simulink model "Copy_of_bike_model_2states_smithFullBike"  (R2018b)
settings: Solver=VariableStepAuto  StartTime=0.0  StopTime=sim_time  FixedStep=Ts/10  MaxStep=Ts/10
values from neighbouring files (symbols this model uses):
  A_bike = [0 g/h_real ; 1 0]    [configuration.m]
  B_bike = [1 ; 0]    [configuration.m]
  b_compFilter = 1.095    [configuration.m]    (also in configuration_pidTuning.m)
  b_real = 1.095    [configuration.m]    (also in configuration_pidTuning.m)
  C1_bike = a_real/(b_real*h_real)    (= 0.392543973584)    [configuration.m]
  C2_bike = 1/(b_real*h_real)    (= 1.15454109878)    [configuration.m]
  C_ini = [C1_bike*input_velocity C2_bike*input_velocity^2]    [configuration.m]
  complementary = 0.985    [configuration.m]    (also in configuration_pidTuning.m)
  D = zeros(3,1)    [configuration_pidTuning.m]
  D_steering_position = 0.0    (= 0)    [configuration.m]
  delay_tf_steering = 0    [configuration.m]
  den_tf_steering = [1 245.9 0]    [configuration.m]
  den_tf_steering_dis = [den_tf_steering_dis 0] - [0 den_tf_steering_dis]    [configuration.m]
  direct_control = 1    [configuration.m]    (also in configuration_pidTuning.m)
  f_filter_phidot = 20    [configuration.m]
  filter_model = 1    [configuration.m]    (also in configuration_pidTuning.m)
  forward_motor_dynamics = 0    [configuration.m]    (also in configuration_pidTuning.m)
  forward_speed_offset = 0    [configuration.m]
  g = 9.81    [configuration.m]    (also in configuration_pidTuning.m)
  I_direct = 0.000227125326188444    (= 0.000227125326188)    [configuration.m]    (also in configuration_pidTuning.m)
  I_lat = 0.000115580509653549    (= 0.000115580509654)    [configuration.m]    (also in configuration_pidTuning.m)
  I_steering_position = 1    [configuration.m]    (also in simulate_bike.m = 30)
  IMU_height_model = 0.45    [configuration.m]    (also in configuration_pidTuning.m)
  IMU_height_real = 0.45    [configuration.m]    (also in configuration_pidTuning.m)
  initial_states = [deg2rad(-2) deg2rad(0) deg2rad(0)]    [configuration.m]    (also in configuration_pidTuning.m)
  input_velocity = 4    [configuration.m]    (also in configuration_pidTuning.m = 3)
  K_fullbike = 1    [configuration.m]
  lambda_compFilter = deg2rad(70)    [configuration.m]    (also in configuration_pidTuning.m)
  lambda_real = deg2rad(70)    [configuration.m]    (also in configuration_pidTuning.m)
  lat_control = 0    [configuration.m]    (also in configuration_pidTuning.m = 1)
  look_ahead = 0    [configuration.m]    (also in configuration_pidTuning.m)
  lqr_gains = zeros(length(velocity_lqr),1+size(A_bike,1))    [lqr_design.m]
  max_roll = pi/2    (= 1.57079632679)    [configuration.m]    (also in configuration_pidTuning.m)
  max_steering_motor_speed = 0.9    [configuration.m]    (also in configuration_pidTuning.m = 7.5)
  min_roll = - max_roll    (= -1.57079632679)    [configuration.m]    (also in configuration_pidTuning.m)
  min_steering_motor_speed = -0.9    [configuration.m]    (also in configuration_pidTuning.m = -7.5)
  noise = 0    [configuration.m]    (also in configuration_pidTuning.m)
  noise_acc = 2.4869e-05    [configuration.m]    (also in configuration_pidTuning.m)
  noise_encoder = 1e-7    (= 1e-07)    [configuration.m]    (also in configuration_pidTuning.m)
  noise_gyro = 0.005    [configuration.m]    (also in configuration_pidTuning.m = 0.0022)
  noise_hall = 0.0031    [configuration.m]    (also in configuration_pidTuning.m)
  noise_pos_meas = 0    [configuration.m]    (also in configuration_pidTuning.m = 0.51)
  num_tf_steering = [253.4]    [configuration.m]
  num_tf_steering_dis = [num_tf_steering_dis 0]    [configuration.m]
  offset_acc = 0.0*g    (= 0)    [configuration.m]
  offset_encoder = deg2rad(1)    [configuration.m]
  offset_gyro = deg2rad(0)    [configuration.m]
  offset_hall = 0.0    (= 0)    [configuration.m]
  offset_pos_x = 0    [configuration.m]
  offset_pos_y = 0    [configuration.m]
  P_direct = 0.0712859744206787    (= 0.0712859744207)    [configuration.m]    (also in configuration_pidTuning.m)
  P_lat = 0.0465435246389258    (= 0.0465435246389)    [configuration.m]    (also in configuration_pidTuning.m)
  P_steering_position = 10    [configuration.m]    (also in simulate_bike.m = 30)
  parameters_compFilter = [g h_compFilter b_compFilter a_compFilter lambda_compFilter c_compFilter]    [configuration.m]    (also in configuration_pidTuning.m)
  roll_rate_coef = 0.9    [configuration.m]    (also in configuration_pidTuning.m)
  sensor_offset = 0    [configuration.m]
  smith_fullbike = 1    [configuration.m]
  smith_steering = 0    [configuration.m]
  steering_angle_correction = deg2rad(0)    [configuration.m]
  sys_con = ss(A_lqr,B_lqr,C_lqr,D_lqr)    [lqr_design.m]
  time_offset_acc = 7    [configuration.m]
  time_offset_encoder = 10    [configuration.m]
  time_offset_gyro = 7    [configuration.m]
  time_offset_hall = 7    [configuration.m]
  time_offset_pos_x = 7    [configuration.m]
  time_offset_pos_y = 7    [configuration.m]
  Ts = 0.01    [configuration.m]    (also in configuration_pidTuning.m = 0.04)
  Ts_IMU = 0.01    [configuration.m]    (also in configuration_pidTuning.m = 0.04)
  velocity_lqr = [input_velocity - 0.1 , input_velocity , input_velocity + 0.1]    [lqr_design.m]
undefined symbols (not defined in the file or in its folder): A, B, cumulative_dist_along_path, curvature, den_filter_phidot, initial_x, initial_y, num_filter_phidot, path_x, path_y
libraries: simulink x14, simulink_extras x3, dspsigops x2
(part 1 of 3)
settings Model: Creator=Boaz Ash  LastModifiedBy=maximef
settings DebuggingCC: UnconnectedInputMsg=none  UnconnectedOutputMsg=none  UnconnectedLineMsg=none  LibraryContextMissingDiagnostic=none
settings SFSimCC: SimUseLocalCustomCode=off
settings RTWCC: RTWUseLocalCustomCode=off

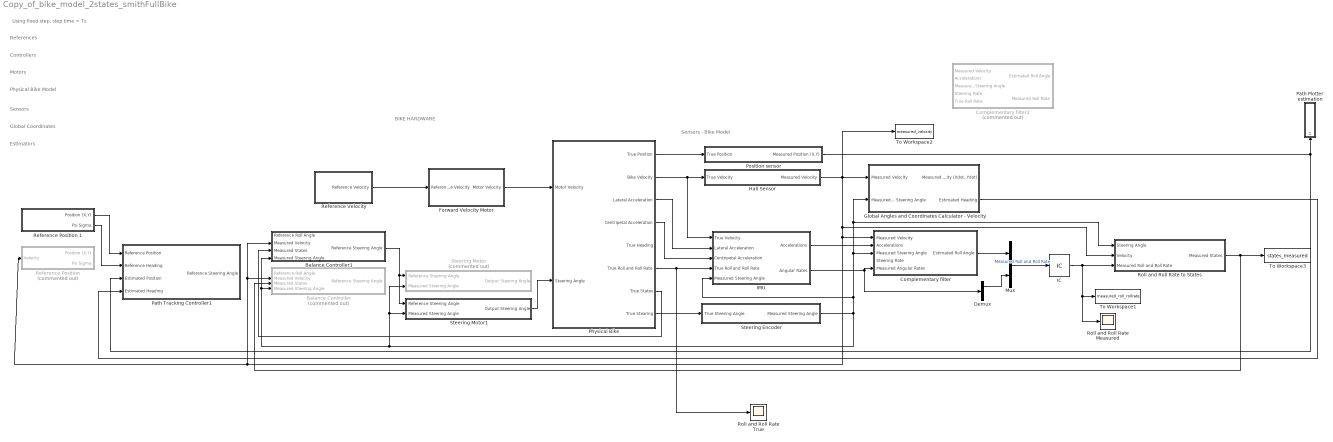
== system Copy_of_bike_model_2states_smithFullBike ==
  note: Using fixed step, step time = Ts
  note: BIKE HARDWARE
  note: References
  note: Physical Bike
      | Model
  note: Sensors - Bike Model
  note: Motors
  note: Sensors
  note: Global Coordinates
  note: Controllers
  note: Estimators
  Balance Controller : Subsystem  Commented=on  TreatAsAtomicUnit=on  SystemSampleTime=Ts
  Balance Controller1 : Subsystem  SystemSampleTime=Ts
  Complementary filter : Subsystem  SystemSampleTime=Ts_IMU
      settings: MinAlgLoopOccurrences=on
  Complementary filter2 : Subsystem  Commented=on  SystemSampleTime=Ts_IMU
      settings: MinAlgLoopOccurrences=on
  Demux : Demux  Outputs=3
  Forward Velocity Motor : Subsystem
  Global Angles and Coordinates Calculator - Velocity : Subsystem  SystemSampleTime=Ts
  Hall Sensor : Subsystem  TreatAsAtomicUnit=on  SystemSampleTime=Ts
  IC : InitialCondition  Value=[initial_states(1) initial_states(3)]'
  IMU : Subsystem  TreatAsAtomicUnit=on
  Mux : Mux  Inputs=2
  Path Plotter estimation : Subsystem  SystemSampleTime=Ts
  Path Tracking Controller1 : Subsystem
  Physical Bike : Subsystem
  Position sensor : Subsystem  TreatAsAtomicUnit=on  SystemSampleTime=Ts
  "Reference Position " : Subsystem  Commented=on
  Reference Position 1 : Subsystem
  "Reference Velocity " : Subsystem
  Roll and Roll Rate Measured : Scope
  Roll and Roll Rate True : Scope
  Roll and Roll Rate to States : Subsystem
  Steering Encoder : Subsystem  TreatAsAtomicUnit=on  SystemSampleTime=Ts
  Steering Motor : Subsystem  Commented=on
  Steering Motor1 : Subsystem
  To Workspace1 : ToWorkspace  VariableName=measured_roll_rollrate  SaveFormat=Timeseries  SampleTime=-1
  To Workspace2 : ToWorkspace  VariableName=measured_velocity  SaveFormat=Timeseries  SampleTime=-1
  To Workspace3 : ToWorkspace  VariableName=states_measured  SaveFormat=Timeseries  SampleTime=-1
  wires:
  "Reference Velocity "/1(Reference Velocity) -> Forward Velocity Motor/1(Reference Velocity)
  Forward Velocity Motor/1(Motor Velocity) -> Physical Bike/1(Motor Velocity)
  Position sensor/1("Measured Position (X,Y) ") -> Path Plotter estimation/1(Position), Path Tracking Controller1/3(Estimated Position)
  Global Angles and Coordinates Calculator - Velocity/2(Estimated Heading) -> Path Tracking Controller1/4(Estimated Heading)
  Physical Bike/3(Lateral Acceleration) -> IMU/2(Lateral Acceleration)
  Physical Bike/4(Centripetal Acceleration) -> IMU/3(Centripetal Acceleration)
  Steering Encoder/1(Measured Steering Angle) -> Steering Motor1/2(Measured Steering Angle), Steering Motor/2(Measured Steering Angle), Balance Controller1/4(Measured Steering Angle), Balance Controller/4(Measured Steering Angle), Roll and Roll Rate to States/1(Steering Angle), Global Angles and Coordinates Calculator - Velocity/2("Measured Steering Angle "), Complementary filter/3(Measured Steering Angle), IMU/5(Measured Steering Angle)
  IMU/1(Accelerations) -> Complementary filter/2(Accelerations)
  Hall Sensor/1(Measured Velocity) -> "Reference Position "/1(Velocity), Balance Controller1/2(Measured Velocity), Balance Controller/2(Measured Velocity), Complementary filter/1(Measured Velocity), Roll and Roll Rate to States/2(Velocity), To Workspace2/1, Global Angles and Coordinates Calculator - Velocity/1(Measured Velocity)
  Reference Position 1/2(Psi Sigma) -> Path Tracking Controller1/2(Reference Heading)
  Reference Position 1/1(Position (X,Y)) -> Path Tracking Controller1/1(Reference Position)
  Physical Bike/1(True Position) -> Position sensor/1(True Position)
  IMU/2(Angular Rates) -> Demux/1, Complementary filter/5(Measured Angular Rates)
  Physical Bike/8(True Stearing) -> Steering Encoder/1(True Steering Angle)
  Physical Bike/6(True Roll and Roll Rate) -> Roll and Roll Rate True/1, IMU/4(True Roll and Roll Rate)
  Physical Bike/2(Bike Velocity) -> IMU/1(True Velocity), Hall Sensor/1(True Velocity)
  IC/1 -> Roll and Roll Rate to States/3(Measured Roll and Roll Rate), Roll and Roll Rate Measured/1, To Workspace1/1
  Mux/1 -> IC/1  "Measured Roll and Roll Rate"
  Complementary filter/1(Estimated Roll Angle) -> Mux/1
  Demux/1 -> Mux/2
  Roll and Roll Rate to States/1(Measured States) -> Balance Controller/3(Measured States), To Workspace3/1
  Balance Controller1/1(Reference Steering Angle) -> Steering Motor1/1(Reference Steering Angle), Steering Motor/1(Reference Steering Angle)
  Physical Bike/7(True States) -> Balance Controller1/3(Measured States)
  Steering Motor1/1(Output Steering Angle) -> Physical Bike/2(Steering Angle)

== system Copy_of_bike_model_2states_smithFullBike/Balance Controller ==
  Reference Roll Angle : Inport
  Measured Velocity : Inport  Port=2
  Measured States : Inport  Port=3
  Measured Steering Angle : Inport  Port=4
  LQR Controller : Subsystem  TreatAsAtomicUnit=on  SystemSampleTime=Ts
  Mux : Mux  Inputs=2
  Reference States Generator : Subsystem  SystemSampleTime=Ts
  Sum : Sum  Inputs=|+-
  To Workspace : ToWorkspace  VariableName=states_measured  SaveFormat=Timeseries  SampleTime=-1
  Reference Steering Angle : Outport
  wires:
  Measured Velocity/1 -> LQR Controller/1(Velocity), Reference States Generator/1(Velocity)
  Measured States/1 -> To Workspace/1, Sum/2
  Measured Steering Angle/1 -> Reference States Generator/2(Steering Angle)
  Reference States Generator/1(State Error) -> LQR Controller/2(State Error)
  Sum/1 -> Reference States Generator/3(Angles Error)
  Mux/1 -> Sum/1
  Reference Roll Angle/1 -> Mux/1
  LQR Controller/1(Calculated Input) -> Reference Steering Angle/1

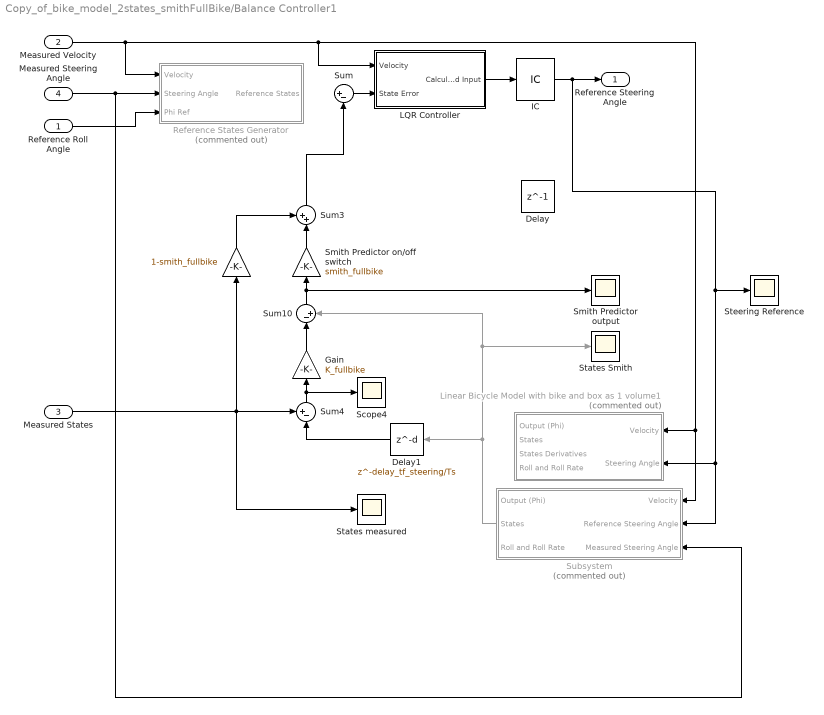
== system Copy_of_bike_model_2states_smithFullBike/Balance Controller1 ==
  Reference Roll Angle : Inport
  Measured Velocity : Inport  Port=2
  Measured States : Inport  Port=3
  Measured Steering Angle : Inport  Port=4
  " " : Gain  Gain=1-smith_fullbike
  Delay : Delay  DelayLength=1
  Delay1 : Delay  DelayLength=delay_tf_steering/Ts  SampleTime=Ts
  Gain : Gain  Gain=K_fullbike
  IC : InitialCondition  Value=0
  LQR Controller : Subsystem  TreatAsAtomicUnit=on  SystemSampleTime=Ts
  Linear Bicycle Model with bike and box as 1 volume1 : Subsystem  Commented=on
  Reference States Generator : Subsystem  Commented=on  SystemSampleTime=Ts
  Scope4 : Scope
  Smith Predictor on/off switch : Gain  Gain=smith_fullbike
  Smith Predictor output : Scope
  States Smith : Scope
  States measured : Scope
  Steering Reference : Scope
  Subsystem : Subsystem  Commented=on
  Sum : Sum  Inputs=|+-
  Sum10 : Sum  Inputs=|-+
  Sum3 : Sum  Inputs=++|
  Sum4 : Sum  Inputs=+-|
  Reference Steering Angle : Outport
  wires:
  Sum/1 -> LQR Controller/2(State Error)
  LQR Controller/1(Calculated Input) -> IC/1
  Reference Roll Angle/1 -> Reference States Generator/3(Phi Ref)
  Measured Steering Angle/1 -> Subsystem/3(Measured Steering Angle), Reference States Generator/2(Steering Angle)
  Measured States/1 -> " "/1, States measured/1, Sum4/1
  " "/1 -> Sum3/1
  Sum3/1 -> Sum/2
  Subsystem/2(States) -> Sum10/2, States Smith/1, Delay1/1
  Gain/1 -> Sum10/1
  Delay1/1 -> Sum4/2
  Smith Predictor on/off switch/1 -> Sum3/2
  Sum10/1 -> Smith Predictor output/1, Smith Predictor on/off switch/1
  Sum4/1 -> Scope4/1, Gain/1
  IC/1 -> Linear Bicycle Model with bike and box as 1 volume1/2(Steering Angle), Subsystem/2(Reference Steering Angle), Steering Reference/1, Reference Steering Angle/1
  Measured Velocity/1 -> Linear Bicycle Model with bike and box as 1 volume1/1(Velocity), Subsystem/1("Velocity "), LQR Controller/1(Velocity), Reference States Generator/1(Velocity)

== system Copy_of_bike_model_2states_smithFullBike/Complementary filter ==
  Measured Velocity : Inport
  Accelerations : Inport  Port=2
  Measured Steering Angle : Inport  Port=3
  Steering Rate : Inport  Port=4
  Measured Angular Rates : Inport  Port=5
  Complementary Filter : Subsystem  TreatAsAtomicUnit=on  SystemSampleTime=Ts_IMU
  Delay4 : Delay  DelayLength=1  SampleTime=Ts_IMU
  Demux : Demux  Outputs=3
  Downsample : DownSample  N=Ts/Ts_IMU  RateOptions=Allow multirate processing
  Roll Angle Estimation of Accelerometer : Subsystem
  To Workspace1 : ToWorkspace  VariableName=IMU_roll_angle  SaveFormat=Structure  SampleTime=-1
  Estimated Roll Angle : Outport
  wires:
  Roll Angle Estimation of Accelerometer/1(Roll Angle Estimation of Accelerometer) -> Complementary Filter/1(Roll Angle Estimation due to Accelerometer)  "Roll_acc"
  Complementary Filter/1(Roll Angle Estimation) -> Downsample/1, Delay4/1
  Measured Velocity/1 -> Roll Angle Estimation of Accelerometer/3(Measured Velocity)
  Measured Steering Angle/1 -> Roll Angle Estimation of Accelerometer/2(Measured Steering Angle)
  Steering Rate/1 -> Roll Angle Estimation of Accelerometer/4(Steering Rate)
  Demux/1 -> Roll Angle Estimation of Accelerometer/5(Roll Rate), Complementary Filter/2(Roll Rate due to Gyroscope)
  Accelerations/1 -> Roll Angle Estimation of Accelerometer/1(Accelerations)
  Measured Angular Rates/1 -> Demux/1
  Delay4/1 -> Roll Angle Estimation of Accelerometer/6(Measured Roll Angle)
  Downsample/1 -> Estimated Roll Angle/1, To Workspace1/1

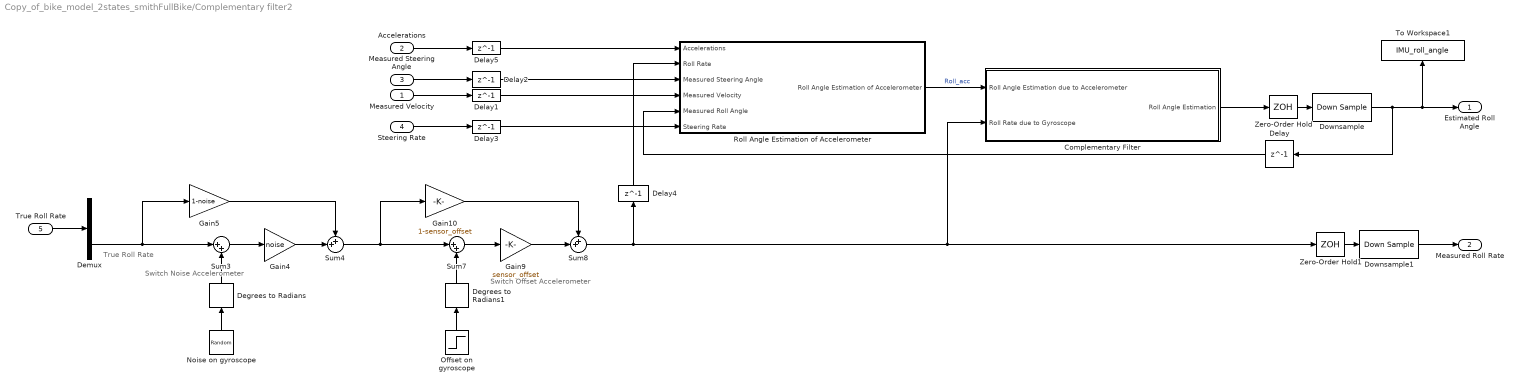
== system Copy_of_bike_model_2states_smithFullBike/Complementary filter2 ==
  note: Switch Noise
      | Accelerometer
  note: True Roll
      | Rate
  note: Switch Offset
      | Accelerometer
  Measured Velocity : Inport
  Accelerations : Inport  Port=2
  Measured Steering Angle : Inport  Port=3
  Steering Rate : Inport  Port=4
  True Roll Rate : Inport  Port=5
  Complementary Filter : Subsystem  TreatAsAtomicUnit=on  SystemSampleTime=Ts_IMU
  Degrees to Radians : simulink_extras/Transformations/Degrees to Radians
  Degrees to Radians1 : simulink_extras/Transformations/Degrees to Radians
  Delay{,1..2,4..5} (5 alike) : Delay  DelayLength=1
  Delay3 : Delay  DelayLength=1  SampleTime=Ts_IMU
  Demux : Demux  Outputs=2
  Downsample : DownSample  N=Ts/Ts_IMU  RateOptions=Allow multirate processing
  Downsample1 : DownSample  N=Ts/Ts_IMU  RateOptions=Allow multirate processing
  Gain10 : Gain  Gain=1-sensor_offset
  Gain4 : Gain  Gain=noise
  Gain5 : Gain  Gain=1-noise
  Gain9 : Gain  Gain=sensor_offset
  Noise on gyroscope : RandomNumber  Variance=noise_gyro  SampleTime=Ts
  Offset on gyroscope : Step  Time=time_offset_gyro  After=offset_gyro  SampleTime=Ts
  Roll Angle Estimation of Accelerometer : Subsystem
  Sum3 : Sum  Inputs=|++
  Sum4 : Sum  Inputs=++|
  Sum7 : Sum  Inputs=|++
  Sum8 : Sum  Inputs=++|
  To Workspace1 : ToWorkspace  VariableName=IMU_roll_angle  SaveFormat=Structure  SampleTime=-1
  Zero-Order Hold : ZeroOrderHold  SampleTime=Ts_IMU
  Zero-Order Hold1 : ZeroOrderHold  SampleTime=Ts_IMU
  Estimated Roll Angle : Outport
  Measured Roll Rate : Outport  Port=2
  wires:
  Roll Angle Estimation of Accelerometer/1(Roll Angle Estimation of Accelerometer) -> Complementary Filter/1(Roll Angle Estimation due to Accelerometer)  "Roll_acc"
  Sum8/1 -> Zero-Order Hold1/1, Complementary Filter/2(Roll Rate due to Gyroscope), Delay4/1
  Zero-Order Hold/1 -> Downsample/1
  Zero-Order Hold1/1 -> Downsample1/1
  Accelerations/1 -> Delay5/1
  Measured Steering Angle/1 -> Delay2/1
  Measured Velocity/1 -> Delay1/1
  Delay/1 -> Roll Angle Estimation of Accelerometer/5(Measured Roll Angle)
  Delay1/1 -> Roll Angle Estimation of Accelerometer/4(Measured Velocity)
  Delay2/1 -> Roll Angle Estimation of Accelerometer/3(Measured Steering Angle)
  Steering Rate/1 -> Delay3/1
  Delay3/1 -> Roll Angle Estimation of Accelerometer/6(Steering Rate)
  Delay4/1 -> Roll Angle Estimation of Accelerometer/2(Roll Rate)
  Delay5/1 -> Roll Angle Estimation of Accelerometer/1(Accelerations)
  Complementary Filter/1(Roll Angle Estimation) -> Zero-Order Hold/1
  Downsample1/1 -> Measured Roll Rate/1
  Downsample/1 -> Estimated Roll Angle/1, To Workspace1/1, Delay/1
  Demux/2 -> Gain5/1, Sum3/1
  Sum3/1 -> Gain4/1
  Noise on gyroscope/1 -> Degrees to Radians/1
  Gain4/1 -> Sum4/2
  Gain5/1 -> Sum4/1
  Degrees to Radians/1 -> Sum3/2
  True Roll Rate/1 -> Demux/1
  Gain9/1 -> Sum8/2
  Sum7/1 -> Gain9/1
  Sum4/1 -> Gain10/1, Sum7/1
  Degrees to Radians1/1 -> Sum7/2
  Offset on gyroscope/1 -> Degrees to Radians1/1
  Gain10/1 -> Sum8/1

== system Copy_of_bike_model_2states_smithFullBike/Forward Velocity Motor ==
  note: Add limit for acceleration/deceleration
      | Add min speed of 1.69 m/s (3600 rpm motor speed) limitation
      | Add min speed of 8.20 m/s (18000 rpm motor speed) limitation
      | Add deadband and delay
  Reference Velocity : Inport
  Band-Limited White Noise : simulink/Sources/Band-Limited White Noise  Cov=[0.001]  Ts=Ts  seed=[23341]
  Constant : Constant  Value=forward_motor_dynamics
  Rate Limiter : RateLimiter  RisingSlewLimit=inf  FallingSlewLimit=-inf  SampleTimeMode=inherited
  Saturation : Saturate  UpperLimit=inf  LowerLimit=0
  Sum : Sum  Inputs=|++
  Switch : Switch  Criteria=u2 > Threshold
  Transfer Fcn : TransferFcn  Numerator=[-0.2156 0.556]  Denominator=[1 1.675 0.5558]
  Motor Velocity : Outport
  wires:
  Reference Velocity/1 -> Transfer Fcn/1, Switch/3
  Transfer Fcn/1 -> Rate Limiter/1
  Switch/1 -> Sum/1
  Constant/1 -> Switch/2
  Saturation/1 -> Switch/1
  Rate Limiter/1 -> Saturation/1
  Sum/1 -> Motor Velocity/1

== system Copy_of_bike_model_2states_smithFullBike/Global Angles and Coordinates Calculator - Velocity ==
  Measured Velocity : Inport
  "Measured Steering Angle " : Inport  Port=2
  Gain1 : Gain  Gain=sin(lambda_compFilter)
  Measured Bike Angles to Global Angles : Subsystem
  Measured Global Angles to Global Coordinates : Subsystem
  Sum : Sum  Inputs=++|
  "Measured Velocity (Xdot, Ydot)" : Outport
  Estimated Heading : Outport  Port=2
  wires:
  "Measured Steering Angle "/1 -> Gain1/1
  Measured Bike Angles to Global Angles/1(Psi) -> Sum/2, Measured Global Angles to Global Coordinates/2(Psi)
  Gain1/1 -> Measured Bike Angles to Global Angles/2(Measured Steering Angle)
  Sum/1 -> Estimated Heading/1
  Measured Bike Angles to Global Angles/2(Beta) -> Measured Global Angles to Global Coordinates/3(Beta), Sum/1
  Measured Velocity/1 -> Measured Bike Angles to Global Angles/1(Velocity), Measured Global Angles to Global Coordinates/1(Velocity)
  Measured Global Angles to Global Coordinates/1("Velocity (Xdot, Ydot)") -> "Measured Velocity (Xdot, Ydot)"/1

== system Copy_of_bike_model_2states_smithFullBike/Hall Sensor ==
  note: Switch Noise
  note: Switch Offset
  True Velocity : Inport
  Gain1 : Gain  Gain=noise
  Gain2 : Gain  Gain=1-noise
  Gain3 : Gain  Gain=sensor_offset
  Gain4 : Gain  Gain=1-sensor_offset
  Noise on hall sensor : RandomNumber  Variance=noise_hall  SampleTime=Ts
  Offset : Constant  Value=forward_speed_offset
  Offset on hall sensor : Step  Time=time_offset_hall  After=offset_hall  SampleTime=Ts
  Saturate Signal : Switch  Criteria=u2 > Threshold
  Sum : Sum  Inputs=++|
  Sum1 : Sum  Inputs=|++
  Sum2 : Sum  Inputs=++|
  Sum3 : Sum  Inputs=|++
  Sum4 : Sum  Inputs=++|
  To Workspace3 : ToWorkspace  VariableName=vel_meas  SaveFormat=Timeseries  SampleTime=-1
  Velocity Lower Bound : simulink/Model Verification/Check Static  Lower Bound  Description=0.6 <= u  min=0.6  min_included=on  enabled=on  stopWhenAssertionFail=off  export=on  icon=graphic
      settings: SourceProductName=Simulink
  Zero : Constant  Value=0
  Zero-Order Hold : ZeroOrderHold  SampleTime=Ts
  Measured Velocity : Outport
  wires:
  Sum3/1 -> Saturate Signal/1, Velocity Lower Bound/1
  Noise on hall sensor/1 -> Sum/1
  Zero/1 -> Saturate Signal/3
  Velocity Lower Bound/1 -> Saturate Signal/2
  True Velocity/1 -> Gain2/1, Sum/2
  Gain1/1 -> Sum1/1
  Gain2/1 -> Sum1/2
  Sum/1 -> Gain1/1
  Sum1/1 -> Gain4/1, Sum2/2
  Sum2/1 -> Gain3/1
  Gain4/1 -> Sum3/2
  Gain3/1 -> Sum3/1
  Offset on hall sensor/1 -> Sum2/1
  Sum4/1 -> Zero-Order Hold/1
  Offset/1 -> Sum4/1
  Saturate Signal/1 -> Sum4/2
  Zero-Order Hold/1 -> To Workspace3/1, Measured Velocity/1

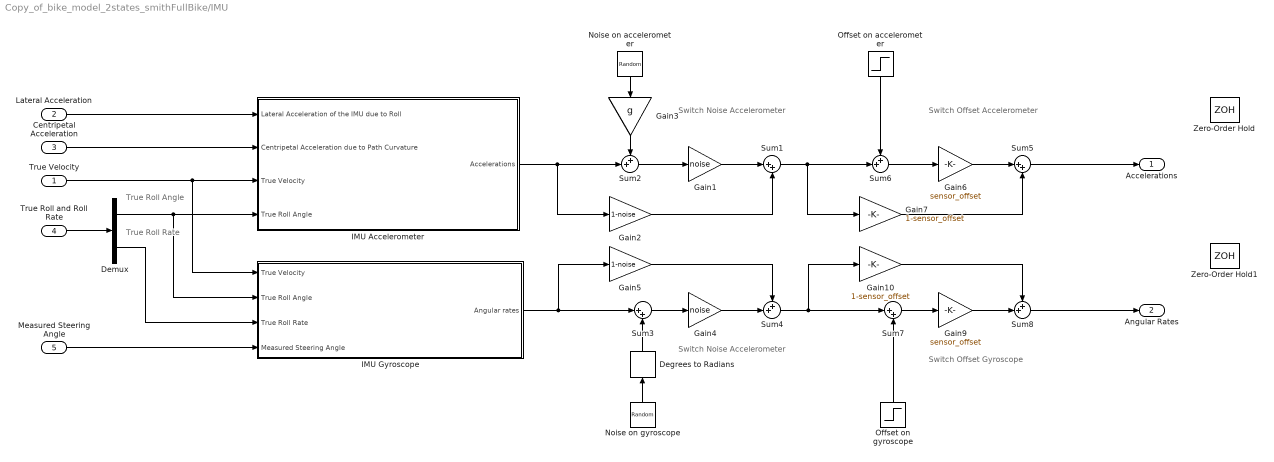
== system Copy_of_bike_model_2states_smithFullBike/IMU ==
  note: True Roll
      | Angle
  note: Switch Noise
      | Accelerometer
  note: Switch Noise
      | Accelerometer
  note: Switch Offset
      | Accelerometer
  note: Switch Offset
      | Gyroscope
  note: True Roll
      | Rate
  True Velocity : Inport
  Lateral Acceleration : Inport  Port=2
  Centripetal Acceleration : Inport  Port=3
  True Roll and Roll Rate : Inport  Port=4
  Measured Steering Angle : Inport  Port=5
  Degrees to Radians : simulink_extras/Transformations/Degrees to Radians
  Demux : Demux  Outputs=2
  Gain1 : Gain  Gain=noise
  Gain10 : Gain  Gain=1-sensor_offset
  Gain2 : Gain  Gain=1-noise
  Gain3 : Gain  Gain=g
  Gain4 : Gain  Gain=noise
  Gain5 : Gain  Gain=1-noise
  Gain6 : Gain  Gain=sensor_offset
  Gain7 : Gain  Gain=1-sensor_offset
  Gain9 : Gain  Gain=sensor_offset
  IMU Accelerometer : Subsystem
  IMU Gyroscope : Subsystem
  Noise on accelerometer : RandomNumber  Variance=noise_acc  SampleTime=Ts
  Noise on gyroscope : RandomNumber  Variance=noise_gyro  SampleTime=Ts
  Offset on accelerometer : Step  Time=time_offset_acc  After=offset_acc  SampleTime=Ts
  Offset on gyroscope : Step  Time=time_offset_gyro  After=offset_gyro  SampleTime=Ts
  Sum{1,3,5,7} (4 alike) : Sum  Inputs=|++
  Sum{2,4,6,8} (4 alike) : Sum  Inputs=++|
  Zero-Order Hold : ZeroOrderHold  SampleTime=Ts_IMU
  Zero-Order Hold1 : ZeroOrderHold  SampleTime=Ts_IMU
  Accelerations : Outport
  Angular Rates : Outport  Port=2
  wires:
  Measured Steering Angle/1 -> IMU Gyroscope/4(Measured Steering Angle)
  True Velocity/1 -> IMU Gyroscope/1(True Velocity), IMU Accelerometer/3(True Velocity)
  Lateral Acceleration/1 -> IMU Accelerometer/1(Lateral Acceleration of the IMU due to Roll)
  Centripetal Acceleration/1 -> IMU Accelerometer/2(Centripetal Acceleration due to Path Curvature)
  True Roll and Roll Rate/1 -> Demux/1
  Demux/1 -> IMU Gyroscope/2(True Roll Angle), IMU Accelerometer/4(True Roll Angle)
  Gain2/1 -> Sum1/2
  IMU Accelerometer/1(Accelerations) -> Sum2/2, Gain2/1
  Noise on accelerometer/1 -> Gain3/1
  Gain3/1 -> Sum2/1
  Noise on gyroscope/1 -> Degrees to Radians/1
  IMU Gyroscope/1(Angular rates) -> Sum3/1, Gain5/1
  Degrees to Radians/1 -> Sum3/2
  Gain5/1 -> Sum4/1
  Sum3/1 -> Gain4/1
  Gain4/1 -> Sum4/2
  Sum2/1 -> Gain1/1
  Gain1/1 -> Sum1/1
  Gain10/1 -> Sum8/1
  Sum4/1 -> Sum7/1, Gain10/1
  Offset on gyroscope/1 -> Sum7/2
  Sum7/1 -> Gain9/1
  Sum6/1 -> Gain6/1
  Offset on accelerometer/1 -> Sum6/1
  Sum1/1 -> Sum6/2, Gain7/1
  Gain6/1 -> Sum5/1
  Gain9/1 -> Sum8/2
  Gain7/1 -> Sum5/2
  Demux/2 -> IMU Gyroscope/3(True Roll Rate)
  Sum5/1 -> Accelerations/1
  Sum8/1 -> Angular Rates/1

== system Copy_of_bike_model_2states_smithFullBike/Path Plotter estimation ==
  Position : Inport
  Demux : Demux  Outputs=2
  To Workspace : ToWorkspace  VariableName=X_BIKE_estim  SaveFormat=Timeseries  SampleTime=Ts
  To Workspace1 : ToWorkspace  VariableName=Y_BIKE_estim  SaveFormat=Timeseries  SampleTime=Ts
  XY Graph : simulink/Sinks/XY Graph  Commented=on  xmin=min(path_x)-5  xmax=max(path_x)+5  ymin=min(path_y)-5  ymax=max(path_y)+5  st=-1
  wires:
  Demux/1 -> XY Graph/1, To Workspace/1  "X"
  Demux/2 -> XY Graph/2, To Workspace1/1  "Y"
  Position/1 -> Demux/1

== system Copy_of_bike_model_2states_smithFullBike/Path Tracking Controller1 ==
  note: Direction Control
  note: Lateral Control
  note: Steering Control
  note: Switch Direct Control
  note: Switch Lateral Control
  Reference Position : Inport
  Reference Heading : Inport  Port=2
  Estimated Position : Inport  Port=3
  Estimated Heading : Inport  Port=4
  " " : Sum  Inputs=|-+
  Gain1 : Gain  Gain=lat_control
  Gain2 : Gain  Gain=direct_control
  Gain3 : Gain  Gain=1-direct_control
  Lateral Error : Subsystem  SystemSampleTime=Ts
  PID Control Lateral Position : simulink/Continuous/PID Controller  Controller=PI  Form=Parallel  TimeDomain=Discrete-time  SampleTime=Ts  IntegratorMethod=Forward Euler  FilterMethod=Forward Euler  ControllerParametersSource=internal  P=P_lat  I=I_lat  D=0  UseFilter=on  N=100  TunerSelectOption=Transfer Function Based (PID Tuner App)  InitialConditionSource=internal  InitialConditionForIntegrator=0  InitialConditionForFilter=0  DifferentiatorICPrevScaledInput=0  ExternalReset=none  TrackingMode=off  Kt=1  LimitOutput=off  UpperSaturationLimit=inf  LowerSaturationLimit=-inf  LinearizeAsGain=on  AntiWindupMode=none  Kb=1  POutMin=[]  POutMax=[]  IOutMin=[]  IOutMax=[]  DOutMin=[]  DOutMax=[]  NOutMin=[]  NOutMax=[]  SumOutMin=[]  SumOutMax=[]  SaturationOutMin=[]  SaturationOutMax=[]  PParamMin=[]  PParamMax=[]  IParamMin=[]  IParamMax=[]  DParamMin=[]  DParamMax=[]  NParamMin=[]  NParamMax=[]  KbParamMin=[]  KbParamMax=[]  KtParamMin=[]  KtParamMax=[]  KbOutMin=[]  KbOutMax=[]  KtOutMin=[]  KtOutMax=[]  IntegratorOutMin=[]  IntegratorOutMax=[]  FilterOutMin=[]  FilterOutMax=[]  SumI1OutMin=[]  SumI1OutMax=[]  SumI2OutMin=[]  SumI2OutMax=[]  SumI3OutMin=[]  SumI3OutMax=[]  SumI4OutMin=[]  SumI4OutMax=[]  SumDOutMin=[]  SumDOutMax=[]  DifferentiatorOutMin=[]  DifferentiatorOutMax=[]  FilterDiffOutCoefMin=[]  FilterDiffOutCoefMax=[]  ReciprocalOutMin=[]  ReciprocalOutMax=[]  SumDenOutMin=[]  SumDenOutMax=[]  SumNumOutMin=[]  SumNumOutMax=[]  DivideOutMin=[]  DivideOutMax=[]  IntegratorContinuousStateAttributes=''  IntegratorStateMustResolveToSignalObject=off  IntegratorRTWStateStorageClass=Auto  FilterContinuousStateAttributes=''  FilterStateMustResolveToSignalObject=off  FilterRTWStateStorageClass=Auto  ParallelPVariant=InternalParameters  IdealPVariant=Disabled  IVariant=InternalParameters  DVariant=Disabled  IntegratorVariant=Discrete  SatVariant=Disabled  AWVariant=Passthrough  PCopyVariant=Disabled  TRVariant=Disabled  FdbkBlocksVariant=Forward  IdealPFdbkVariant=Disabled  SatFdbkVariant=Disabled  DerivativeFilterVariant=Disabled  NVariant=Disabled  NCopyVariant=Disabled_SignalSpec  FilterICVariant=Disabled  IntegratorICVariant=InternalICs  ExternalResetVariant=Disabled  TRSumVariant=Passthrough  SumFdbkVariant=Disabled  SumVariant=Sum_PI
  PID Control Direction : simulink/Continuous/PID Controller  Controller=PI  Form=Parallel  TimeDomain=Discrete-time  SampleTime=Ts  IntegratorMethod=Forward Euler  FilterMethod=Forward Euler  ControllerParametersSource=internal  P=P_direct  I=I_direct  D=0  UseFilter=on  N=100  TunerSelectOption=Transfer Function Based (PID Tuner App)  InitialConditionSource=internal  InitialConditionForIntegrator=0  InitialConditionForFilter=0  DifferentiatorICPrevScaledInput=0  ExternalReset=none  TrackingMode=off  Kt=1  LimitOutput=off  UpperSaturationLimit=inf  LowerSaturationLimit=-inf  LinearizeAsGain=on  AntiWindupMode=none  Kb=1  POutMin=[]  POutMax=[]  IOutMin=[]  IOutMax=[]  DOutMin=[]  DOutMax=[]  NOutMin=[]  NOutMax=[]  SumOutMin=[]  SumOutMax=[]  SaturationOutMin=[]  SaturationOutMax=[]  PParamMin=[]  PParamMax=[]  IParamMin=[]  IParamMax=[]  DParamMin=[]  DParamMax=[]  NParamMin=[]  NParamMax=[]  KbParamMin=[]  KbParamMax=[]  KtParamMin=[]  KtParamMax=[]  KbOutMin=[]  KbOutMax=[]  KtOutMin=[]  KtOutMax=[]  IntegratorOutMin=[]  IntegratorOutMax=[]  FilterOutMin=[]  FilterOutMax=[]  SumI1OutMin=[]  SumI1OutMax=[]  SumI2OutMin=[]  SumI2OutMax=[]  SumI3OutMin=[]  SumI3OutMax=[]  SumI4OutMin=[]  SumI4OutMax=[]  SumDOutMin=[]  SumDOutMax=[]  DifferentiatorOutMin=[]  DifferentiatorOutMax=[]  FilterDiffOutCoefMin=[]  FilterDiffOutCoefMax=[]  ReciprocalOutMin=[]  ReciprocalOutMax=[]  SumDenOutMin=[]  SumDenOutMax=[]  SumNumOutMin=[]  SumNumOutMax=[]  DivideOutMin=[]  DivideOutMax=[]  IntegratorContinuousStateAttributes=''  IntegratorStateMustResolveToSignalObject=off  IntegratorRTWStateStorageClass=Auto  FilterContinuousStateAttributes=''  FilterStateMustResolveToSignalObject=off  FilterRTWStateStorageClass=Auto  ParallelPVariant=InternalParameters  IdealPVariant=Disabled  IVariant=InternalParameters  DVariant=Disabled  IntegratorVariant=Discrete  SatVariant=Disabled  AWVariant=Passthrough  PCopyVariant=Disabled  TRVariant=Disabled  FdbkBlocksVariant=Forward  IdealPFdbkVariant=Disabled  SatFdbkVariant=Disabled  DerivativeFilterVariant=Disabled  NVariant=Disabled  NCopyVariant=Disabled_SignalSpec  FilterICVariant=Disabled  IntegratorICVariant=InternalICs  ExternalResetVariant=Disabled  TRSumVariant=Passthrough  SumFdbkVariant=Disabled  SumVariant=Sum_PI
  Sum1 : Sum  Inputs=|++
  Sum4 : Sum  Inputs=+--
  Reference Steering Angle : Outport
  wires:
  Lateral Error/1(Lateral Error) -> PID Control Lateral Position/1  "Lateral Error"
  Estimated Position/1 -> " "/2
  " "/1 -> Lateral Error/2(Position Error (X,Y))  "Position Error"
  Sum4/1 -> PID Control Direction/1  "Delta Reference = Psi Sigma - Nu"
  Estimated Heading/1 -> Sum4/3
  Gain1/1 -> Gain3/1, Sum4/2
  PID Control Lateral Position/1 -> Gain1/1
  Reference Heading/1 -> Lateral Error/1(Psi Sigma), Sum4/1
  Reference Position/1 -> " "/1
  PID Control Direction/1 -> Gain2/1
  Gain2/1 -> Sum1/1
  Gain3/1 -> Sum1/2
  Sum1/1 -> Reference Steering Angle/1

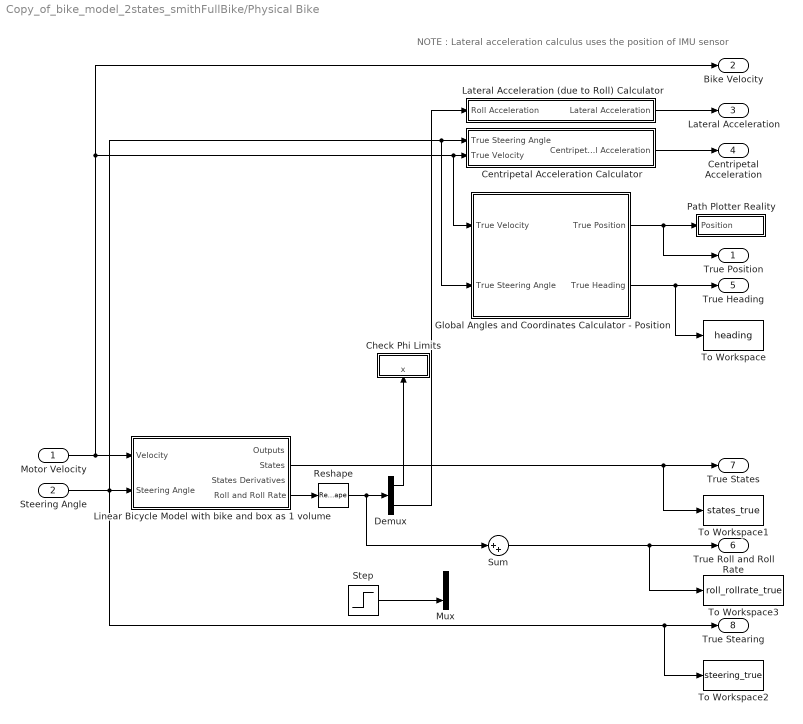
== system Copy_of_bike_model_2states_smithFullBike/Physical Bike ==
  note: NOTE : Lateral acceleration calculus uses the position of IMU sensor
  Motor Velocity : Inport
  Steering Angle : Inport  Port=2
  Centripetal Acceleration Calculator : Subsystem
  Check Phi Limits : Subsystem  TreatAsAtomicUnit=on  SystemSampleTime=Ts
  Demux : Demux  Outputs=2
  Global Angles and Coordinates Calculator - Position : Subsystem  SystemSampleTime=Ts
  Lateral Acceleration (due to Roll) Calculator : Subsystem
  Linear Bicycle Model with bike and box as 1 volume : Subsystem
  Mux : Mux  Inputs=2
  Path Plotter Reality : Subsystem  SystemSampleTime=Ts
  Reshape : Reshape
  Step : Step  Time=10  After=deg2rad(3)  SampleTime=0
  Sum : Sum  Inputs=|++
  To Workspace : ToWorkspace  VariableName=heading  SaveFormat=Timeseries  SampleTime=-1
  To Workspace1 : ToWorkspace  VariableName=states_true  SaveFormat=Timeseries  SampleTime=-1
  To Workspace2 : ToWorkspace  VariableName=steering_true  SaveFormat=Timeseries  SampleTime=-1
  To Workspace3 : ToWorkspace  VariableName=roll_rollrate_true  SaveFormat=Timeseries  SampleTime=-1
  True Position : Outport
  Bike Velocity : Outport  Port=2
  Lateral Acceleration : Outport  Port=3
  Centripetal Acceleration : Outport  Port=4
  True Heading : Outport  Port=5
  True Roll and Roll Rate : Outport  Port=6
  True States : Outport  Port=7
  True Stearing : Outport  Port=8
  wires:
  Steering Angle/1 -> Global Angles and Coordinates Calculator - Position/2(True Steering Angle), Centripetal Acceleration Calculator/1(True Steering Angle), To Workspace2/1, True Stearing/1, Linear Bicycle Model with bike and box as 1 volume/2(Steering Angle)
  Centripetal Acceleration Calculator/1(Centripetal Acceleration) -> Centripetal Acceleration/1
  Lateral Acceleration (due to Roll) Calculator/1(Lateral Acceleration) -> Lateral Acceleration/1
  Motor Velocity/1 -> Global Angles and Coordinates Calculator - Position/1(True Velocity), Centripetal Acceleration Calculator/2(True Velocity), Bike Velocity/1, Linear Bicycle Model with bike and box as 1 volume/1(Velocity)
  Linear Bicycle Model with bike and box as 1 volume/2(States) -> To Workspace1/1, True States/1
  Global Angles and Coordinates Calculator - Position/1(True Position) -> True Position/1, Path Plotter Reality/1(Position)
  Global Angles and Coordinates Calculator - Position/2(True Heading) -> To Workspace/1, True Heading/1
  Demux/2 -> Lateral Acceleration (due to Roll) Calculator/1(Roll Acceleration)
  Demux/1 -> Check Phi Limits/1(x)
  Reshape/1 -> Demux/1, Sum/1
  Linear Bicycle Model with bike and box as 1 volume/4(Roll and Roll Rate) -> Reshape/1
  Sum/1 -> To Workspace3/1, True Roll and Roll Rate/1
  Step/1 -> Mux/2

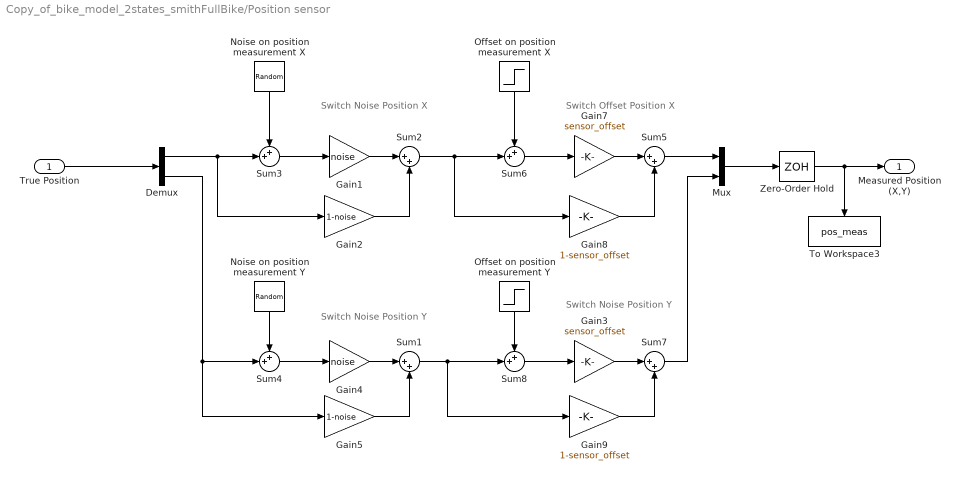
== system Copy_of_bike_model_2states_smithFullBike/Position sensor ==
  note: Switch Noise
      | Position X
  note: Switch Noise
      | Position Y
  note: Switch Offset
      | Position X
  note: Switch Noise
      | Position Y
  True Position : Inport
  Demux : Demux  Outputs=2
  Gain1 : Gain  Gain=noise
  Gain2 : Gain  Gain=1-noise
  Gain3 : Gain  Gain=sensor_offset
  Gain4 : Gain  Gain=noise
  Gain5 : Gain  Gain=1-noise
  Gain7 : Gain  Gain=sensor_offset
  Gain8 : Gain  Gain=1-sensor_offset
  Gain9 : Gain  Gain=1-sensor_offset
  Mux : Mux  Inputs=2
  "Noise on position measurement X    " : RandomNumber  Variance=noise_pos_meas  Seed=2  SampleTime=Ts
  "Noise on position measurement Y     " : RandomNumber  Variance=noise_pos_meas  SampleTime=Ts
  "Offset on position measurement X    " : Step  Time=time_offset_pos_x  After=offset_pos_x  SampleTime=Ts
  "Offset on position measurement Y     " : Step  Time=time_offset_pos_y  After=offset_pos_y  SampleTime=Ts
  Sum{1..2,5,7} (4 alike) : Sum  Inputs=|++
  Sum{3..4,6,8} (4 alike) : Sum  Inputs=++|
  To Workspace3 : ToWorkspace  VariableName=pos_meas  SaveFormat=Timeseries  SampleTime=-1
  Zero-Order Hold : ZeroOrderHold  SampleTime=Ts
  "Measured Position (X,Y) " : Outport
  wires:
  Zero-Order Hold/1 -> To Workspace3/1, "Measured Position (X,Y) "/1
  True Position/1 -> Demux/1
  Mux/1 -> Zero-Order Hold/1
  "Noise on position measurement X    "/1 -> Sum3/1
  Demux/1 -> Gain2/1, Sum3/2
  "Noise on position measurement Y     "/1 -> Sum4/1
  Demux/2 -> Sum4/2, Gain5/1
  Sum3/1 -> Gain1/1
  Gain1/1 -> Sum2/1
  Gain4/1 -> Sum1/1
  Sum4/1 -> Gain4/1
  Gain2/1 -> Sum2/2
  Gain5/1 -> Sum1/2
  Sum2/1 -> Sum6/2, Gain8/1
  "Offset on position measurement X    "/1 -> Sum6/1
  Sum6/1 -> Gain7/1
  Gain8/1 -> Sum5/2
  Gain7/1 -> Sum5/1
  Sum5/1 -> Mux/1
  Gain3/1 -> Sum7/1
  Sum8/1 -> Gain3/1
  "Offset on position measurement Y     "/1 -> Sum8/1
  Sum1/1 -> Gain9/1, Sum8/2
  Gain9/1 -> Sum7/2
  Sum7/1 -> Mux/2

== system Copy_of_bike_model_2states_smithFullBike/Reference Position  ==
  Velocity : Inport
  Add : Sum
  Constant : Constant  Value=look_ahead
  Constant Look Ahead Time : Gain  Gain=0.2
  Integrator2 : Integrator
  Look Ahead Switch : Switch  Criteria=u2 > Threshold
  Mux{,2..4} (4 alike) : Mux  Inputs=2
  Reference Position and Angle Selector : Subsystem
  Scope1 : Scope  NumInputPorts=3
  Subsystem1 : Subsystem
  To Workspace2 : ToWorkspace  VariableName=X_SIGMA  SaveFormat=Timeseries  SampleTime=Ts
  To Workspace3 : ToWorkspace  VariableName=Y_SIGMA  SaveFormat=Timeseries  SampleTime=Ts
  To Workspace5 : ToWorkspace  VariableName=PSI_S  SaveFormat=Timeseries  SampleTime=Ts
  Variable Look Ahead Distance : ManualSwitch
  Variable Look Ahead : Subsystem
  Position (X,Y) : Outport
  Psi Sigma : Outport  Port=2
  wires:
  Constant Look Ahead Time/1 -> Variable Look Ahead Distance/1
  Reference Position and Angle Selector/3(psi_sigma) -> To Workspace5/1, Mux4/2, Psi Sigma/1
  Mux3/1 -> Scope1/1
  Subsystem1/3(psi_sigma) -> Mux4/1
  Mux2/1 -> Scope1/2
  Mux4/1 -> Scope1/3
  Velocity/1 -> Integrator2/1, Constant Look Ahead Time/1, Variable Look Ahead/1(Velocity)
  Add/1 -> Look Ahead Switch/1
  Reference Position and Angle Selector/2(Y_sigma) -> To Workspace3/1, Mux2/2, Mux/2
  Look Ahead Switch/1 -> Reference Position and Angle Selector/1(total travelled distance)
  Subsystem1/2(Y_sigma) -> Mux2/1
  Integrator2/1 -> Variable Look Ahead/2(Total Tavelled Distance), Look Ahead Switch/3, Subsystem1/1(total travelled distance), Add/2  "total travelled distance"
  Subsystem1/1(X_sigma) -> Mux3/1
  Reference Position and Angle Selector/1(X_sigma) -> Mux3/2, To Workspace2/1, Mux/1
  Variable Look Ahead Distance/1 -> Add/1  "Look-Ahead Distance"
  Constant/1 -> Look Ahead Switch/2
  Mux/1 -> Position (X,Y)/1
  Variable Look Ahead/1(Look Ahead Distance) -> Variable Look Ahead Distance/2

== system Copy_of_bike_model_2states_smithFullBike/Reference Position 1 ==
  Mux : Mux  Inputs=2
  Ramp : simulink/Sources/Ramp  slope=3  start=0  InitialOutput=0
  Step : Step  Time=25  After=0.1  SampleTime=0
  Step1 : Step  Time=25  After=deg2rad(0)  SampleTime=0
  To Workspace2 : ToWorkspace  VariableName=X_SIGMA  SaveFormat=Timeseries  SampleTime=Ts
  To Workspace3 : ToWorkspace  VariableName=Y_SIGMA  SaveFormat=Timeseries  SampleTime=Ts
  To Workspace5 : ToWorkspace  VariableName=PSI_S  SaveFormat=Timeseries  SampleTime=Ts
  Position (X,Y) : Outport
  Psi Sigma : Outport  Port=2
  wires:
  Mux/1 -> Position (X,Y)/1
  Ramp/1 -> To Workspace2/1, Mux/1
  Step/1 -> Mux/2, To Workspace3/1
  Step1/1 -> To Workspace5/1, Psi Sigma/1

== system Copy_of_bike_model_2states_smithFullBike/Reference Velocity  ==
  note: If you will use this variable velocity
      | reference generator, you need to change
      | upper and lower limits of velocity specified
      | in initialization code!
  Add : Sum  Inputs=4
  Constant Velocity : Constant  Value=input_velocity
  Ramp : simulink/Sources/Ramp  slope=0.03  start=0  InitialOutput=0
  Reference Velocity Selector : ManualSwitch
  Sine Wave : Sin  Amplitude=0  SampleTime=0
  Step : Step  Time=20  Before=4  After=8  SampleTime=0
  Step1 : Step  Time=40  After=-1  SampleTime=0
  Reference Velocity : Outport
  wires:
  Ramp/1 -> Add/4
  Constant Velocity/1 -> Reference Velocity Selector/1
  Step1/1 -> Add/3
  Step/1 -> Add/2
  Sine Wave/1 -> Add/1
  Add/1 -> Reference Velocity Selector/2
  Reference Velocity Selector/1 -> Reference Velocity/1

== system Copy_of_bike_model_2states_smithFullBike/Roll and Roll Rate to States ==
  Steering Angle : Inport
  Velocity : Inport  Port=2
  Measured Roll and Roll Rate : Inport  Port=3
  Constant1 : Constant  Value=zeros(size(C_ini,1),size(B_bike,2))
  Constant2 : Constant  Value=A_bike
  Constant4 : Constant  Value=B_bike
  Gain : Gain  Gain=C2_bike
  Gain1 : Gain  Gain=C1_bike
  Matrix Concatenate2 : Concatenate  Mode=Multidimensional array
  Matrix Concatenate3 : Concatenate  Mode=Multidimensional array
  Mux2 : Mux  Inputs=2
  Product{1,3..5,9} (5 alike) : Product  SCDEnableBlockLinearizationSpecification=on  Multiplication=Matrix(*)
  Product2 : Product  SCDEnableBlockLinearizationSpecification=on  Inputs=/  Multiplication=Matrix(*)
  Reshape : Reshape  OutputDimensionality=Row vector (2-D)
  Square1 : Math  Operator=square  SaturateOnIntegerOverflow=on
  Sum1 : Sum  Inputs=-+|
  Zero-Order Hold : ZeroOrderHold  SampleTime=Ts
  Measured States : Outport
  wires:
  Reshape/1 -> Product5/1, Matrix Concatenate2/1, Product1/1  "C"
  Velocity/1 -> Square1/1, Gain1/1
  Square1/1 -> Gain/1
  Gain/1 -> Mux2/2
  Gain1/1 -> Mux2/1
  Mux2/1 -> Reshape/1
  Constant2/1 -> Product1/2
  Matrix Concatenate2/1 -> Product2/1  "[C ; CA]"
  Product1/1 -> Matrix Concatenate2/2  "CA"
  Product2/1 -> Product4/1, Product3/1  "inv([C ; CA])"
  Measured Roll and Roll Rate/1 -> Zero-Order Hold/1
  Product3/1 -> Sum1/2  "inv([C ; CA]) [phi ; phidot]"
  Matrix Concatenate3/1 -> Product4/2  "[0 ; CB]"
  Product5/1 -> Matrix Concatenate3/2  "CB"
  Constant4/1 -> Product5/2
  Constant1/1 -> Matrix Concatenate3/1
  Product4/1 -> Product9/1  "inv([C ; CA]) [0 ; CB]"
  Steering Angle/1 -> Product9/2
  Product9/1 -> Sum1/1  "inv([C ; CA]) [0 ; CB] u"
  Sum1/1 -> Measured States/1
  Zero-Order Hold/1 -> Product3/2

== system Copy_of_bike_model_2states_smithFullBike/Steering Encoder ==
  note: Switch Noise
  note: True Steering
      | Angle
  note: Switch Offset
  True Steering Angle : Inport
  Gain1 : Gain  Gain=noise
  Gain2 : Gain  Gain=1-noise
  Gain3 : Gain  Gain=sensor_offset
  Gain4 : Gain  Gain=1-sensor_offset
  Noise on steering encoder : RandomNumber  Variance=noise_encoder  Seed=6  SampleTime=Ts
  Offset correction : Constant  Value=steering_angle_correction
  Offset on steering encoder : Step  Time=time_offset_encoder  After=offset_encoder  SampleTime=Ts
  Sum : Sum  Inputs=++|
  Sum1 : Sum  Inputs=|++
  Sum2 : Sum  Inputs=+++
  Sum3 : Sum  Inputs=++|
  Sum4 : Sum  Inputs=|++
  Zero-Order Hold : ZeroOrderHold  SampleTime=Ts
  Measured Steering Angle : Outport
  wires:
  Sum/1 -> Gain1/1
  Noise on steering encoder/1 -> Sum/1
  True Steering Angle/1 -> Gain2/1, Sum/2
  Gain2/1 -> Sum1/2
  Gain1/1 -> Sum1/1
  Sum2/1 -> Zero-Order Hold/1
  Zero-Order Hold/1 -> Measured Steering Angle/1
  Gain3/1 -> Sum4/1
  Sum1/1 -> Gain4/1, Sum3/2
  Offset on steering encoder/1 -> Sum3/1
  Sum3/1 -> Gain3/1
  Gain4/1 -> Sum4/2
  Sum4/1 -> Sum2/2

== system Copy_of_bike_model_2states_smithFullBike/Steering Motor ==
  Reference Steering Angle : Inport
  Measured Steering Angle : Inport  Port=2
  Delay : Delay  DelayLength=delay_tf_steering/Ts  SampleTime=Ts
  Discrete FIR Filter : DiscreteFir  Coefficients=[0.5 0.5]%0.1*ones(10,1)
  Gain : Gain  Gain=1/Ts
  Integrator : Integrator  InitialCondition=initial_states(2)
  Mux : Mux  Inputs=2
  PID Controller : simulink/Continuous/PID Controller  Controller=P  Form=Parallel  TimeDomain=Discrete-time  SampleTime=Ts  IntegratorMethod=Forward Euler  FilterMethod=Forward Euler  ControllerParametersSource=internal  P=P_steering_position  I=0  D=0  UseFilter=off  N=1  TunerSelectOption=Transfer Function Based (PID Tuner App)  InitialConditionSource=internal  InitialConditionForIntegrator=0  InitialConditionForFilter=0  DifferentiatorICPrevScaledInput=0  ExternalReset=none  TrackingMode=off  Kt=1  LimitOutput=off  UpperSaturationLimit=inf  LowerSaturationLimit=-inf  LinearizeAsGain=on  AntiWindupMode=none  Kb=1  POutMin=[]  POutMax=[]  IOutMin=[]  IOutMax=[]  DOutMin=[]  DOutMax=[]  NOutMin=[]  NOutMax=[]  SumOutMin=[]  SumOutMax=[]  SaturationOutMin=[]  SaturationOutMax=[]  PParamMin=[]  PParamMax=[]  IParamMin=[]  IParamMax=[]  DParamMin=[]  DParamMax=[]  NParamMin=[]  NParamMax=[]  KbParamMin=[]  KbParamMax=[]  KtParamMin=[]  KtParamMax=[]  KbOutMin=[]  KbOutMax=[]  KtOutMin=[]  KtOutMax=[]  IntegratorOutMin=[]  IntegratorOutMax=[]  FilterOutMin=[]  FilterOutMax=[]  SumI1OutMin=[]  SumI1OutMax=[]  SumI2OutMin=[]  SumI2OutMax=[]  SumI3OutMin=[]  SumI3OutMax=[]  SumI4OutMin=[]  SumI4OutMax=[]  SumDOutMin=[]  SumDOutMax=[]  DifferentiatorOutMin=[]  DifferentiatorOutMax=[]  FilterDiffOutCoefMin=[]  FilterDiffOutCoefMax=[]  ReciprocalOutMin=[]  ReciprocalOutMax=[]  SumDenOutMin=[]  SumDenOutMax=[]  SumNumOutMin=[]  SumNumOutMax=[]  DivideOutMin=[]  DivideOutMax=[]  IntegratorContinuousStateAttributes=''  IntegratorStateMustResolveToSignalObject=off  IntegratorRTWStateStorageClass=Auto  FilterContinuousStateAttributes=''  FilterStateMustResolveToSignalObject=off  FilterRTWStateStorageClass=Auto  ParallelPVariant=InternalParameters  IdealPVariant=Disabled  IVariant=Disabled  DVariant=Disabled  IntegratorVariant=Disabled  SatVariant=Disabled  AWVariant=Disabled  PCopyVariant=Disabled  TRVariant=Disabled  FdbkBlocksVariant=Forward  IdealPFdbkVariant=Disabled  SatFdbkVariant=Disabled  DerivativeFilterVariant=Disabled  NVariant=Disabled  NCopyVariant=Disabled_SignalSpec  FilterICVariant=Disabled  IntegratorICVariant=Disabled  ExternalResetVariant=Disabled  TRSumVariant=Passthrough  SumFdbkVariant=Disabled  SumVariant=Passthrough_P
  Scope : Scope
  Scope1 : Scope
  Scope2 : Scope
  Steering motor delay1 : Delay  DelayLength=1  SampleTime=Ts
  Steering motor transfer function Steering Rate reference to Steering Rate : TransferFcn  Numerator=[num_tf_steering]  Denominator=[den_tf_steering]
  Sum : Sum  Inputs=|+-
  Sum1 : Sum  Inputs=|-+
  Sum2 : Sum  Inputs=|++
  To Workspace : ToWorkspace  VariableName=calculated_input  SaveFormat=Timeseries  SampleTime=Ts
  To Workspace1 : ToWorkspace  VariableName=realised_input  SaveFormat=Timeseries  SampleTime=-1
  Output Steering Angle : Outport
  wires:
  Mux/1 -> Scope/1
  Steering motor transfer function Steering Rate reference to Steering Rate/1 -> Integrator/1  "Realised Steering Rate"
  Delay/1 -> Steering motor transfer function Steering Rate reference to Steering Rate/1
  PID Controller/1 -> Sum2/1  "Steering Rate Reference"
  Sum/1 -> PID Controller/1
  Reference Steering Angle/1 -> Scope2/1, Mux/1, To Workspace/1, Sum1/2, Steering motor delay1/1, Sum/1  "Realised Steering Angle"
  Gain/1 -> Discrete FIR Filter/1
  Steering motor delay1/1 -> Sum1/1
  Sum1/1 -> Scope1/1, Gain/1
  Sum2/1 -> Delay/1
  Discrete FIR Filter/1 -> Sum2/2
  Integrator/1 -> Output Steering Angle/1, To Workspace1/1, Mux/2  "Realised Steering Angle"
  Measured Steering Angle/1 -> Sum/2
